simulink subsystem "PreChangerCircuit"  (R2023a)
settings: Solver=VariableStepAuto  StartTime=0.0  StopTime=10.0  RelTol=1e-3
undefined symbols (not defined in the file): PlntBattCntctrThresh, PlntBattPreChrgCapParCond, PlntBattPreChrgRes
libraries: fl_lib x8, nesl_utility_internal x8, ee_lib x4
settings Model: Creator=The MathWorks, Inc.  LastModifiedBy=The MathWorks, Inc.
settings SolverCC: AlgebraicLoopSolver=TrustRegion  MaxZcPerStep=1
settings OptimizationCC: ReuseModelBlockBuffer=off
settings DebuggingCC: UnconnectedInputMsg=warning  UnconnectedOutputMsg=warning  UnconnectedLineMsg=warning
settings ModelReferenceCC: EnableRefExpFcnMdlSchedulingChecks=on
settings RTWCC: DLArmComputeVersion=19.05

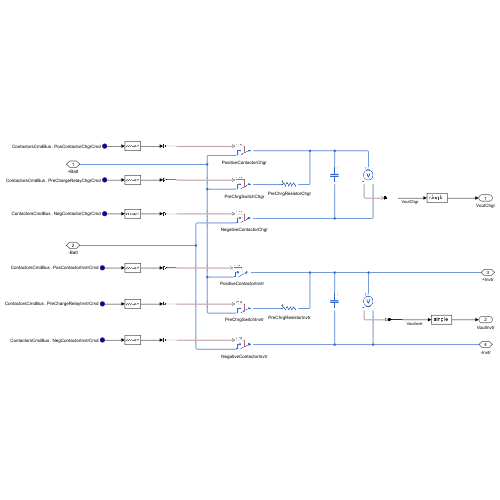
[thumbnail: Simulink's stored preview of the top-level diagram]
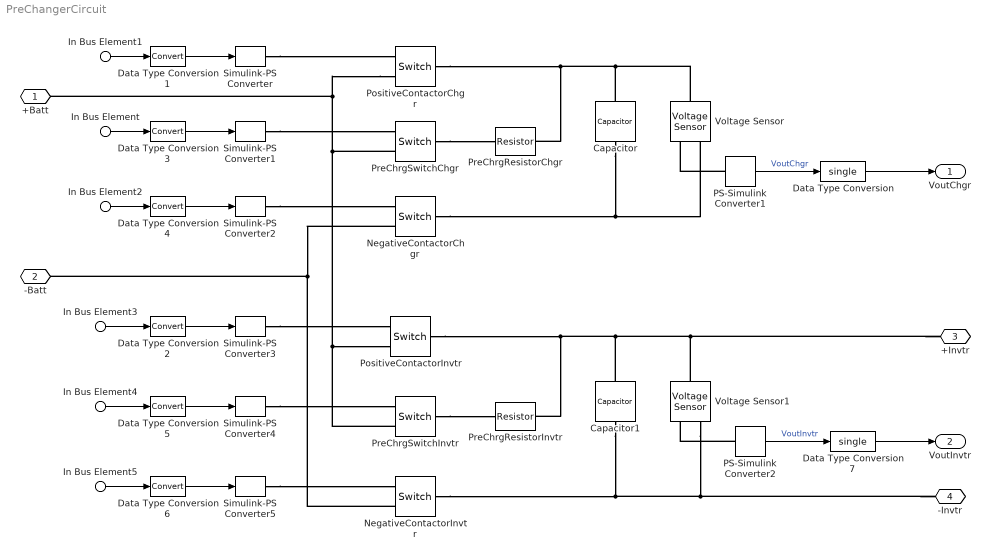
== system PreChangerCircuit ==
  In Bus Element1 : Inport  PortName=ContactorsCmdBus  Element=PosContactorChgrCmd
  In Bus Element : Inport  PortName=ContactorsCmdBus  Element=PreChargeRelayChgrCmd
  In Bus Element2 : Inport  PortName=ContactorsCmdBus  Element=NegContactorChgrCmd
  In Bus Element3 : Inport  PortName=ContactorsCmdBus  Element=PosContactorInvtrCmd
  In Bus Element4 : Inport  PortName=ContactorsCmdBus  Element=PreChargeRelayInvtrCmd
  In Bus Element5 : Inport  PortName=ContactorsCmdBus  Element=NegContactorInvtrCmd
  Capacitor : ee_lib/Passive/Capacitor  cap_option=0  c=PlntBattPreChrgCap uF  Cvec=[1e-05, 1e-06] F  Vvec=[0, 10] V  CV_table_symmetry=1  f_vec=[1, 10] kHz  DFext_vec=[.8, 1.2]  enable_C_tol=0  averaging_period=0 s  C_tol=5  tol_distribution=1  nSigma=4  r=PlntBattPreChrgCapSerRes Ohm  g=PlntBattPreChrgCapParCond 1/Ohm  enable_operating_limits=0  enable_faults=ee.enum.enable.no  fault_action=simscape.enum.assert.action.none  Cscale_faulted=100  R_faulted=1e-3 Ohm  G_faulted=0 1/Ohm  tau_fault=1e-3 s  fault_trigger=ee.enum.faults.faultTrigger.temporal  t_fault=1 s  max_permissible_voltage_range=[-100, 100] V  t_fail_on_voltage=1 s  operating_limit_action=2  max_working_voltage_range=[-25, 25] V  power_rating=1 W  i_specify=off  i_priority=None  i=0 A  i_nominal_specify=off  i_nominal_unit=A  i_nominal_value=1  v_specify=off  v_priority=None  v=0 V  v_nominal_specify=off  v_nominal_unit=V  v_nominal_value=1  vc_specify=off  vc_priority=High  vc=0 V  vc_nominal_specify=off  vc_nominal_unit=V  vc_nominal_value=1
      settings: SourceProductName=Electrical
  Capacitor1 : ee_lib/Passive/Capacitor  cap_option=0  c=PlntBattPreChrgCap uF  Cvec=[1e-05, 1e-06] F  Vvec=[0, 10] V  CV_table_symmetry=1  f_vec=[1, 10] kHz  DFext_vec=[.8, 1.2]  enable_C_tol=0  averaging_period=0 s  C_tol=5  tol_distribution=1  nSigma=4  r=PlntBattPreChrgCapSerRes Ohm  g=PlntBattPreChrgCapParCond 1/Ohm  enable_operating_limits=0  enable_faults=ee.enum.enable.no  fault_action=simscape.enum.assert.action.none  Cscale_faulted=100  R_faulted=1e-3 Ohm  G_faulted=0 1/Ohm  tau_fault=1e-3 s  fault_trigger=ee.enum.faults.faultTrigger.temporal  t_fault=1 s  max_permissible_voltage_range=[-100, 100] V  t_fail_on_voltage=1 s  operating_limit_action=2  max_working_voltage_range=[-25, 25] V  power_rating=1 W  i_specify=off  i_priority=None  i=0 A  i_nominal_specify=off  i_nominal_unit=A  i_nominal_value=1  v_specify=off  v_priority=None  v=0 V  v_nominal_specify=off  v_nominal_unit=V  v_nominal_value=1  vc_specify=off  vc_priority=High  vc=0 V  vc_nominal_specify=off  vc_nominal_unit=V  vc_nominal_value=1
      settings: SourceProductName=Electrical
  Data Type Conversion : DataTypeConversion  OutDataTypeStr=single  SaturateOnIntegerOverflow=off  RndMeth=Floor
  Data Type Conversion{1..6} (6 alike) : DataTypeConversion  SaturateOnIntegerOverflow=off  RndMeth=Floor
  Data Type Conversion7 : DataTypeConversion  OutDataTypeStr=single  SaturateOnIntegerOverflow=off  RndMeth=Floor
  NegativeContactorChgr : fl_lib/Electrical/Electrical Elements/Switch  R_closed=PlntBattCntctrClsdRes Ohm  G_open=PlntBattCntctrOpenCond 1/Ohm  Threshold=PlntBattCntctrThresh  i_specify=off  i_priority=None  i=0 A  i_nominal_specify=off  i_nominal_unit=A  i_nominal_value=1  v_specify=off  v_priority=None  v=0 V  v_nominal_specify=off  v_nominal_unit=V  v_nominal_value=1
      settings: SourceProductName=Foundation Library
  NegativeContactorInvtr : fl_lib/Electrical/Electrical Elements/Switch  R_closed=PlntBattCntctrClsdRes Ohm  G_open=PlntBattCntctrOpenCond 1/Ohm  Threshold=PlntBattCntctrThresh  i_specify=off  i_priority=None  i=0 A  i_nominal_specify=off  i_nominal_unit=A  i_nominal_value=1  v_specify=off  v_priority=None  v=0 V  v_nominal_specify=off  v_nominal_unit=V  v_nominal_value=1
      settings: SourceProductName=Foundation Library
  PS-Simulink Converter1 : nesl_utility_internal/PS-Simulink Converter  PhysicalDomain=network_engine_domain  SubClassName=ps_output  LeftPortType=input  RightPortType=output  PseudoPeriodic=off  Frequencies=[]  VectorFormat=1-D array  Unit=V  AffineConversion=off
  PS-Simulink Converter2 : nesl_utility_internal/PS-Simulink Converter  PhysicalDomain=network_engine_domain  SubClassName=ps_output  LeftPortType=input  RightPortType=output  PseudoPeriodic=off  Frequencies=[]  VectorFormat=1-D array  Unit=V  AffineConversion=off
  PositiveContactorChgr : fl_lib/Electrical/Electrical Elements/Switch  R_closed=PlntBattCntctrClsdRes Ohm  G_open=PlntBattCntctrOpenCond 1/Ohm  Threshold=PlntBattCntctrThresh  i_specify=off  i_priority=None  i=0 A  i_nominal_specify=off  i_nominal_unit=A  i_nominal_value=1  v_specify=off  v_priority=None  v=0 V  v_nominal_specify=off  v_nominal_unit=V  v_nominal_value=1
      settings: SourceProductName=Foundation Library
  PositiveContactorInvtr : fl_lib/Electrical/Electrical Elements/Switch  R_closed=PlntBattCntctrClsdRes Ohm  G_open=PlntBattCntctrOpenCond 1/Ohm  Threshold=PlntBattCntctrThresh  i_specify=off  i_priority=None  i=0 A  i_nominal_specify=off  i_nominal_unit=A  i_nominal_value=1  v_specify=off  v_priority=None  v=0 V  v_nominal_specify=off  v_nominal_unit=V  v_nominal_value=1
      settings: SourceProductName=Foundation Library
  PreChrgResistorChgr : ee_lib/Passive/Resistor  R=PlntBattPreChrgRes Ohm  enable_R_tol=0  R_tol=5  tol_distribution=1  nSigma=4  enable_operating_limits=0  operating_limit_action=2  power_rating=1 W  max_working_voltage=100 V  enable_faults=ee.enum.enable.no  fault_action=simscape.enum.assert.action.none  R_faulted=inf Ohm  fault_trigger=ee.enum.faults.faultTrigger.temporal  t_fault=1 s  max_permissible_current=1 A  t_fail_on_current=1 s  noise_mode=0  Tdevice=25 degC  sample_time=1e-3 s  repeatability=1  user_seed=0  auto_seed=3046698749  power_derating_T1=70 degC  power_derating_T2=155 degC  operating_temperature_range_vec=[-50, 150] degC  alpha=3.93e-3 1/K  Tmeas=25 degC  thermal_mass=100 J/K  temperature_specify=off  temperature_priority=High  temperature=298.15 K  temperature_nominal_specify=off  temperature_nominal_unit=K  temperature_nominal_value=1
      settings: SourceProductName=Electrical
  PreChrgResistorInvtr : ee_lib/Passive/Resistor  R=PlntBattPreChrgRes Ohm  enable_R_tol=0  R_tol=5  tol_distribution=1  nSigma=4  enable_operating_limits=0  operating_limit_action=2  power_rating=1 W  max_working_voltage=100 V  enable_faults=ee.enum.enable.no  fault_action=simscape.enum.assert.action.none  R_faulted=inf Ohm  fault_trigger=ee.enum.faults.faultTrigger.temporal  t_fault=1 s  max_permissible_current=1 A  t_fail_on_current=1 s  noise_mode=0  Tdevice=25 degC  sample_time=1e-3 s  repeatability=1  user_seed=0  auto_seed=3241354618  power_derating_T1=70 degC  power_derating_T2=155 degC  operating_temperature_range_vec=[-50, 150] degC  alpha=3.93e-3 1/K  Tmeas=25 degC  thermal_mass=100 J/K  temperature_specify=off  temperature_priority=High  temperature=298.15 K  temperature_nominal_specify=off  temperature_nominal_unit=K  temperature_nominal_value=1
      settings: SourceProductName=Electrical
  PreChrgSwitchChgr : fl_lib/Electrical/Electrical Elements/Switch  R_closed=PlntBattCntctrClsdRes Ohm  G_open=PlntBattCntctrOpenCond 1/Ohm  Threshold=PlntBattCntctrThresh  i_specify=off  i_priority=None  i=0 A  i_nominal_specify=off  i_nominal_unit=A  i_nominal_value=1  v_specify=off  v_priority=None  v=0 V  v_nominal_specify=off  v_nominal_unit=V  v_nominal_value=1
      settings: SourceProductName=Foundation Library
  PreChrgSwitchInvtr : fl_lib/Electrical/Electrical Elements/Switch  R_closed=PlntBattCntctrClsdRes Ohm  G_open=PlntBattCntctrOpenCond 1/Ohm  Threshold=PlntBattCntctrThresh  i_specify=off  i_priority=None  i=0 A  i_nominal_specify=off  i_nominal_unit=A  i_nominal_value=1  v_specify=off  v_priority=None  v=0 V  v_nominal_specify=off  v_nominal_unit=V  v_nominal_value=1
      settings: SourceProductName=Foundation Library
  Simulink-PS Converter{,1..5} (6 alike) : nesl_utility_internal/Simulink-PS Converter  PhysicalDomain=network_engine_domain  SubClassName=ps_input  LeftPortType=input  RightPortType=output  PseudoPeriodic=off  Frequencies=[]  NoiseDistribution=none  NoiseParameters=[]  Unit=1  AffineConversion=off  FilteringAndDerivatives=provide  SimscapeFilterOrder=1  InputFilterTimeConstant=0.001  UdotUserProvided=0
  Voltage Sensor : fl_lib/Electrical/Electrical Sensors/Voltage Sensor
      settings: SourceProductName=Foundation Library
  Voltage Sensor1 : fl_lib/Electrical/Electrical Sensors/Voltage Sensor
      settings: SourceProductName=Foundation Library
  +Batt : PMIOPort  Side=Left
  -Batt : PMIOPort  Port=2  Side=Left
  +Invtr : PMIOPort  Port=3  Side=Right
  -Invtr : PMIOPort  Port=4  Side=Right
  VoutChgr : Outport  VectorParamsAs1DForOutWhenUnconnected=off
  VoutInvtr : Outport  Port=2  VectorParamsAs1DForOutWhenUnconnected=off
  wires:
  Data Type Conversion6/1 -> Simulink-PS Converter5/1
  In Bus Element4/1 -> Data Type Conversion5/1
  Data Type Conversion7/1 -> VoutInvtr/1
  Data Type Conversion/1 -> VoutChgr/1
  In Bus Element3/1 -> Data Type Conversion2/1
  Data Type Conversion3/1 -> Simulink-PS Converter1/1
  In Bus Element5/1 -> Data Type Conversion6/1
  Data Type Conversion2/1 -> Simulink-PS Converter3/1
  PS-Simulink Converter1/1 -> Data Type Conversion/1  "VoutChgr"
  Data Type Conversion1/1 -> Simulink-PS Converter/1
  Data Type Conversion5/1 -> Simulink-PS Converter4/1
  PS-Simulink Converter2/1 -> Data Type Conversion7/1  "VoutInvtr"
  Data Type Conversion4/1 -> Simulink-PS Converter2/1
  In Bus Element/1 -> Data Type Conversion3/1
  In Bus Element1/1 -> Data Type Conversion1/1
  In Bus Element2/1 -> Data Type Conversion4/1
  connections:
  PreChrgResistorInvtr/RConn1 -- Voltage Sensor1/LConn1 -- +Invtr/RConn1 -- Capacitor1/LConn1 -- PositiveContactorInvtr/LConn1
  PositiveContactorChgr/LConn1 -- Capacitor/LConn1 -- Voltage Sensor/LConn1 -- PreChrgResistorChgr/RConn1
  PositiveContactorChgr/RConn2 -- PositiveContactorInvtr/RConn2 -- PreChrgSwitchInvtr/RConn2 -- PreChrgSwitchChgr/RConn2 -- +Batt/RConn1
  Voltage Sensor/RConn2 -- Capacitor/RConn1 -- NegativeContactorChgr/LConn1
  -Invtr/RConn1 -- Capacitor1/RConn1 -- NegativeContactorInvtr/LConn1 -- Voltage Sensor1/RConn2
  NegativeContactorInvtr/RConn2 -- -Batt/RConn1 -- NegativeContactorChgr/RConn2
  Simulink-PS Converter3/RConn1 -- PositiveContactorInvtr/RConn1
  Simulink-PS Converter2/RConn1 -- NegativeContactorChgr/RConn1
  Simulink-PS Converter1/RConn1 -- PreChrgSwitchChgr/RConn1
  PS-Simulink Converter1/LConn1 -- Voltage Sensor/RConn1
  PreChrgSwitchInvtr/LConn1 -- PreChrgResistorInvtr/LConn1
  PS-Simulink Converter2/LConn1 -- Voltage Sensor1/RConn1
  Simulink-PS Converter/RConn1 -- PositiveContactorChgr/RConn1
  PreChrgSwitchChgr/LConn1 -- PreChrgResistorChgr/LConn1
  Simulink-PS Converter4/RConn1 -- PreChrgSwitchInvtr/RConn1
  Simulink-PS Converter5/RConn1 -- NegativeContactorInvtr/RConn1
